simulink model "lego_SF_MCC"  (Simulink 10.2)
settings: Solver=FixedStepDiscrete  StartTime=0.0  StopTime=Inf  RelTol=1e-3  EnableMultiTasking=on
values from neighbouring files (symbols this model uses):
  Sd = c2d(Sc,Te,'zoh')    [AncienTest.m]    (also in Test.m)
  Te = 1/100    (= 0.01)    [AncienTest.m]    (also in Test.m)
undefined symbols (not defined in the file or in its folder): DiscIntNeverNeededParam, Kd
libraries: simulink x1, rpi_blkst x1
settings Model: Creator=jacques  LastModifiedBy=etudiant  SimulationMode=external
settings DataIOCC: LimitDataPoints=on
settings OptimizationCC: ExpressionDepthLimit=2147483647  LifeSpan=1  EfficientTunableParamExpr=on
settings DebuggingCC: SolverPrmCheckMsg=warning  StateNameClashWarn=warning
settings HardwareCC: ProdIntDivRoundTo=Zero  ProdEndianess=LittleEndian  ProdHWDeviceType=Intel->x86/Pentium
settings SFSimCC: MATLABDynamicMemAlloc=off
settings RTWCC: Description=RTW Embedded Coder RPI target  SystemTargetFile=ert_rpi.tlc  TemplateMakefile=ert_rpi.tmf  PostCodeGenCommand=postGenFunc(buildInfo)
settings CodeAppCC: IgnoreCustomStorageClasses=off  CustomSymbolStrType=$N$R$M  InternalIdentifier=Classic
settings STFCustomTargetCC: ModelReferenceCompliant=off  CombineOutputUpdateFcns=on  ERTCustomFileBanners=on  SupportNonInlinedSFcns=off  RemoveResetFunc=on  MATLABClassNameForMDSCustomization=Simulink.SoftwareTarget.ERTCustomization  GRTInterface=off  SystemTargetFile=ert_rpi.tlc
settings ERTTargetCC: MultiwordLength=2048  ModelReferenceCompliant=off  ParMdlRefBuildCompliant=off  CompOptLevelCompliant=off  ConcurrentExecutionCompliant=off  SupportContinuousTime=on  ModelStepFunctionPrototypeControlCompliant=off  CPPClassGenCompliant=off  UseToolchainInfoCompliant=off  ExtMode=on  ExtModeMexArgs='127.0.0.1'  ERTCustomFileTemplate=ert_rpi_file_process.tlc  ConvertIfToSwitch=off  SuppressUnreachableDefaultCases=off

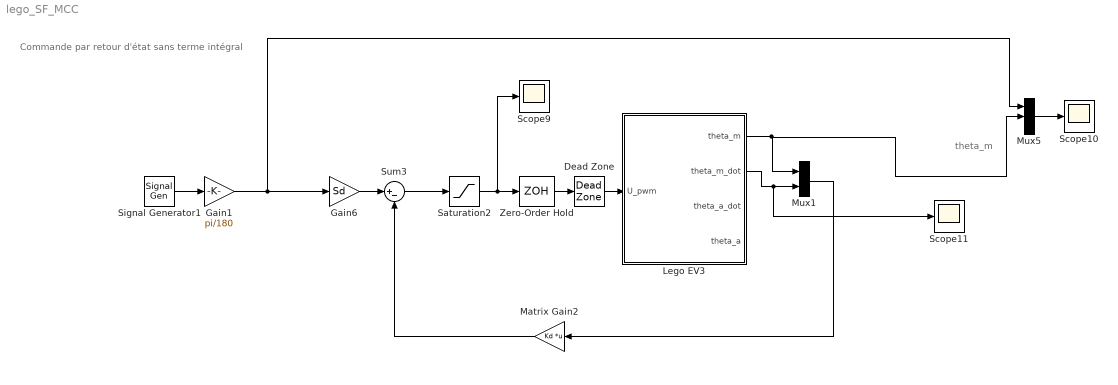
== system lego_SF_MCC ==
  note: Commande par retour d'état sans terme intégral
  note: theta_m
  Dead Zone : DeadZone  LowerValue=-1  UpperValue=1  SaturateOnIntegerOverflow=on
  Gain1 : Gain  Gain=pi/180  SaturateOnIntegerOverflow=on  OutDataTypeStr=Inherit: Same as input  ParamDataTypeStr=Inherit: Same as input
  Gain6 : Gain  Gain=Sd  SaturateOnIntegerOverflow=on  OutDataTypeStr=Inherit: Same as input  ParamDataTypeStr=Inherit: Same as input
  Lego EV3 : Subsystem
  Matrix Gain2 : Gain  Gain=Kd  Multiplication=Matrix(K*u)  SaturateOnIntegerOverflow=on  OutDataTypeStr=Inherit: Same as input  ParamDataTypeStr=Inherit: Same as input
  Mux1 : Mux  Inputs=2
  Mux5 : Mux  Inputs=3
  Saturation2 : Saturate  UpperLimit=100  LowerLimit=-100
  Scope10 : Scope
  Scope11 : Scope
  Scope9 : Scope
  Signal Generator1 : SignalGenerator  WaveForm=square  Amplitude=5  Frequency=0.2
  Sum3 : Sum  Inputs=|+-  SaturateOnIntegerOverflow=on
  Zero-Order Hold : ZeroOrderHold  SampleTime=Te
  wires:
  Zero-Order Hold/1 -> Dead Zone/1
  Matrix Gain2/1 -> Sum3/2
  Gain6/1 -> Sum3/1
  Lego EV3/1(theta_m) -> Mux5/2, Mux1/1
  Saturation2/1 -> Scope9/1, Zero-Order Hold/1
  Mux5/1 -> Scope10/1
  Sum3/1 -> Saturation2/1
  Lego EV3/2(theta_m_dot) -> Scope11/1, Mux1/2
  Signal Generator1/1 -> Gain1/1
  Mux1/1 -> Matrix Gain2/1
  Gain1/1 -> Gain6/1, Mux5/1
  Dead Zone/1 -> Lego EV3/1(U_pwm)

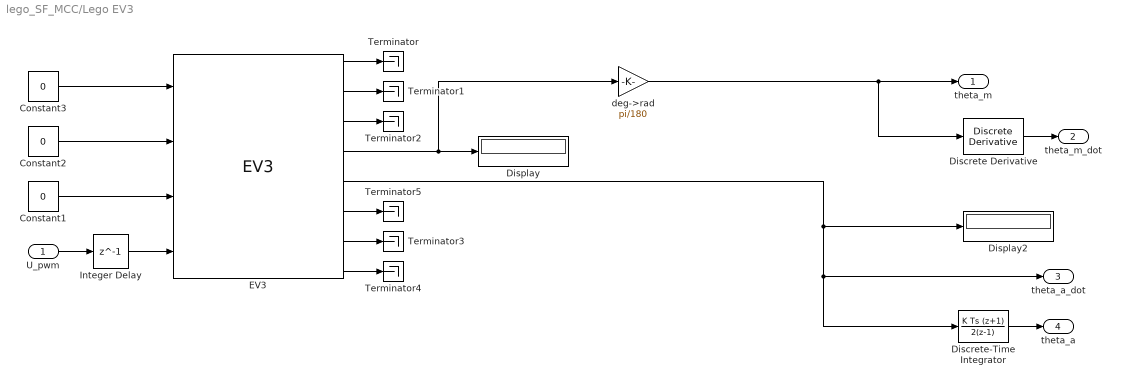
== system lego_SF_MCC/Lego EV3 ==
  U_pwm : Inport
  Constant1 : Constant  Value=0  SampleTime=0.01
  Constant2 : Constant  Value=0  SampleTime=0.01
  Constant3 : Constant  Value=0  SampleTime=0.01
  Discrete Derivative : simulink/Discrete/Discrete Derivative  gainval=1.0  ICPrevScaledInput=0.0  OutMin=[]  OutMax=[]  OutDataType=fixdt(1, 16)  OutScaling=2^-10  DoSatur=off
  Discrete-Time Integrator : DiscreteIntegrator  IntegratorMethod=Integration: Trapezoidal  SampleTime=-1  ICPrevOutput=DiscIntNeverNeededParam  ICPrevScaledInput=DiscIntNeverNeededParam
  Display : Display
  Display2 : Display
  EV3 : rpi_blkst/EV3  rpi_mask_Ts=0.01
      settings: SourceProductName=RPI Blockset
  Integer Delay : Delay  DelayLength=1  SampleTime=0.01
  Terminator{,1..5} (6 alike) : Terminator
  deg->rad : Gain  Gain=pi/180
  theta_m : Outport
  theta_m_dot : Outport  Port=2
  theta_a_dot : Outport  Port=3
  theta_a : Outport  Port=4
  wires:
  U_pwm/1 -> Integer Delay/1
  Constant1/1 -> EV3/3
  Constant2/1 -> EV3/2
  Constant3/1 -> EV3/1
  EV3/1 -> Terminator/1
  EV3/2 -> Terminator1/1
  EV3/3 -> Terminator2/1
  EV3/7 -> Terminator3/1
  EV3/8 -> Terminator4/1
  EV3/4 -> Display/1, deg->rad/1
  EV3/5 -> Display2/1, theta_a_dot/1, Discrete-Time Integrator/1
  Integer Delay/1 -> EV3/4
  deg->rad/1 -> Discrete Derivative/1, theta_m/1
  EV3/6 -> Terminator5/1
  Discrete-Time Integrator/1 -> theta_a/1
  Discrete Derivative/1 -> theta_m_dot/1
